simulink model "unicycle_b_point"  (R2025b)
settings: Solver=ode45  StartTime=0.0  StopTime=40  FixedStep=1e-4  MaxStep=0.01  RelTol=1e-3
settings Model: Creator=Cris  LastModifiedBy=Cris
settings DebuggingCC: UnderspecifiedInitializationDetection=Classic  MergeDetectMultiDrivingBlocksExec=none
settings ModelReferenceCC: PropagateSignalLabelsOutOfModel=off

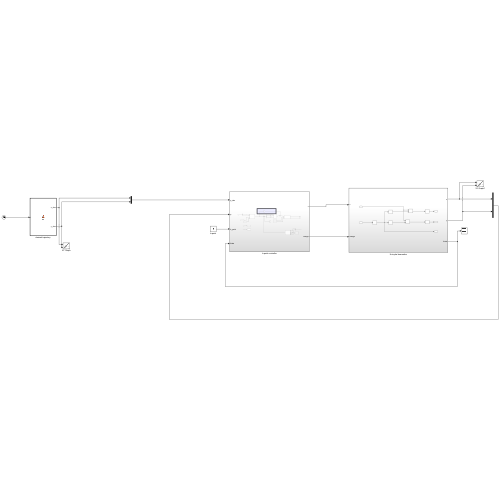
[thumbnail: Simulink's stored preview of the top-level diagram]
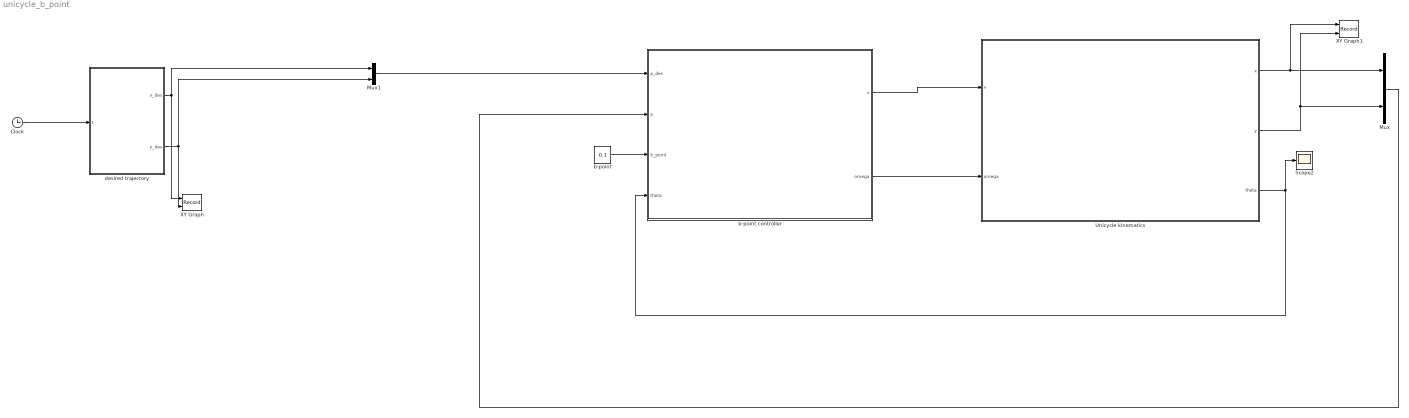
== system unicycle_b_point ==
  Clock : Clock
  Mux : Mux  Inputs=2
  Mux1 : Mux  Inputs=2
  Scope2 : Scope
      settings: ActiveDisplayYMinimum=-1  ActiveDisplayYMaximum=1
  Unicycle kinematics : Subsystem
  XY Graph : Record  NumPorts=2.0  FileSettingsInternal="{\"entries\":[{\"content\":{\"excelSettings\":{\"content\":{},\"type\":\"Streamout.ExcelSettings\"},\"parquetSettings\":{\"content\":{},\"type\":\"Streamout.ParquetSettings\"}},\"type\":\"Streamout.FileSettingStorage\",\"uuid\":\"\"}],\"packageUris\":[\"http:\\/\\/schema.mathworks.com\\/mf0\\/streamout_blocks\\/R2020a\"],\"version\":\"1.0\"}"  FrameSettings=[0, 0]  Layout=[1 1]  SignalsInternal="{\"entries\":[{\"content\":{\"signals\":[{\"content\":{\"blockPath\":[],\"dimensions\":[1],\"domain\":\"\",\"lineColor\":\"#a2142f\",\"plots\":[ 1 ],\"port\":1,\"sid\":[\"\"],\"signalID\":1,\"signalName\":\"desired trajectory:1\"},\"type\":\"RecordBlkView.Signal\",\"uuid\":\"\"},{\"content\":{\"blockPath\":[],\"dimensions\":[1],\"domain\":\"\",\"lineColor\":\"#139fff\",\"plots\":[ 1 ],\"port\":2,\"sid\":[\"\"],\"signalID\":2,\"signalName\":\"desired trajectory:2\"},\"type\":\"RecordBlkView.Signal\",\"uuid\":\"\"}]},\"type\":\"RecordBlkView.InputSignals\",\"uuid\":\"\"}],\"packageUris\":[\"http:\\/\\/schema.mathworks.com\\/mf0\\/streamout_blocks\\/R2020a\"],\"version\":\"1.0\"}"  VisualizationBindings="{\"xyplotplugin\":{\"info\":[{\"series\":[{\"bindingParametersList\":[{\"parameter\":\"X-Axis\",\"signalID\":1,\"signalName\":\"desired trajectory:1\"},{\"parameter\":\"Y-Axis\",\"signalID\":2,\"signalName\":\"desired trajectory:2\"}],\"seriesID\":0}],\"subplotID\":1}]}}"  CompatibilityTag=XY
  XY Graph1 : Record  NumPorts=2.0  FileSettingsInternal="{\"entries\":[{\"content\":{\"excelSettings\":{\"content\":{},\"type\":\"Streamout.ExcelSettings\"},\"parquetSettings\":{\"content\":{},\"type\":\"Streamout.ParquetSettings\"}},\"type\":\"Streamout.FileSettingStorage\",\"uuid\":\"\"}],\"packageUris\":[\"http:\\/\\/schema.mathworks.com\\/mf0\\/streamout_blocks\\/R2020a\"],\"version\":\"1.0\"}"  FrameSettings=[0, 0]  Layout=[1 1]  SignalsInternal="{\"entries\":[{\"content\":{\"signals\":[{\"content\":{\"blockPath\":[],\"dimensions\":[1],\"domain\":\"\",\"lineColor\":\"#a2142f\",\"plots\":[ 1 ],\"port\":1,\"sid\":[\"\"],\"signalID\":1,\"signalName\":\"Unicycle kinematics:1\"},\"type\":\"RecordBlkView.Signal\",\"uuid\":\"\"},{\"content\":{\"blockPath\":[],\"dimensions\":[1],\"domain\":\"\",\"lineColor\":\"#139fff\",\"plots\":[ 1 ],\"port\":2,\"sid\":[\"\"],\"signalID\":2,\"signalName\":\"Unicycle kinematics:2\"},\"type\":\"RecordBlkView.Signal\",\"uuid\":\"\"}]},\"type\":\"RecordBlkView.InputSignals\",\"uuid\":\"\"}],\"packageUris\":[\"http:\\/\\/schema.mathworks.com\\/mf0\\/streamout_blocks\\/R2020a\"],\"version\":\"1.0\"}"  VisualizationBindings="{\"xyplotplugin\":{\"info\":[{\"series\":[{\"bindingParametersList\":[{\"parameter\":\"X-Axis\",\"signalID\":1,\"signalName\":\"Unicycle kinematics:1\"},{\"parameter\":\"Y-Axis\",\"signalID\":2,\"signalName\":\"Unicycle kinematics:2\"}],\"seriesID\":0}],\"subplotID\":1}]}}"  CompatibilityTag=XY
  b-point : Constant  Value=0.1
  b-point controller : Subsystem
  desired trajectory : MATLAB Function  TreatAsAtomicUnit=on
  wires:
  Unicycle kinematics/1(x) -> XY Graph1/1, Mux/1
  Unicycle kinematics/2(y) -> XY Graph1/2, Mux/2
  Unicycle kinematics/3(theta) -> b-point controller/4(theta), Scope2/1
  desired trajectory/1(x_des) -> Mux1/1, XY Graph/1
  desired trajectory/2(y_des) -> Mux1/2, XY Graph/2
  Clock/1 -> desired trajectory/1(t)
  b-point controller/1(v) -> Unicycle kinematics/1(v)
  b-point controller/2(omega) -> Unicycle kinematics/2(omega)
  b-point/1 -> b-point controller/3(b_point)
  Mux1/1 -> b-point controller/1(p_des)
  Mux/1 -> b-point controller/2(p)

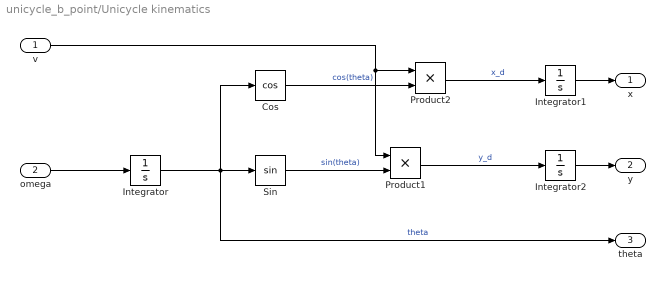
== system unicycle_b_point/Unicycle kinematics ==
  v : Inport
  omega : Inport  Port=2
  Cos : Trigonometry  Operator=cos
  Integrator : Integrator
  Integrator1 : Integrator
  Integrator2 : Integrator
  Product1 : Product
  Product2 : Product
  Sin : Trigonometry
  x : Outport
  y : Outport  Port=2
  theta : Outport  Port=3
  wires:
  omega/1 -> Integrator/1
  Integrator/1 -> theta/1, Cos/1, Sin/1  "theta"
  Cos/1 -> Product2/2  "cos(theta)"
  Sin/1 -> Product1/2  "sin(theta)"
  v/1 -> Product2/1, Product1/1
  Integrator1/1 -> x/1
  Product2/1 -> Integrator1/1  "x_d"
  Integrator2/1 -> y/1
  Product1/1 -> Integrator2/1  "y_d"

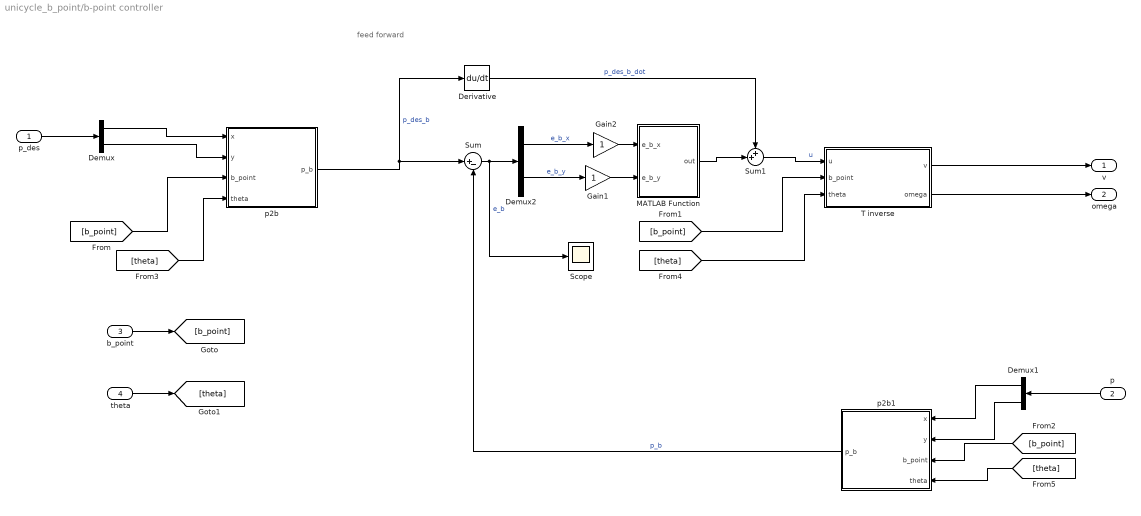
== system unicycle_b_point/b-point controller ==
  note: feed forward
  p_des : Inport
  p : Inport  Port=2
  b_point : Inport  Port=3
  theta : Inport  Port=4
  Demux : Demux  Outputs=2
  Demux1 : Demux  Outputs=2
  Demux2 : Demux  Outputs=2
  Derivative : Derivative
  Gain1 : Gain
  Gain2 : Gain
  MATLAB Function : MATLAB Function  TreatAsAtomicUnit=on
  Scope : Scope
      settings: ActiveDisplayYMinimum=-1  ActiveDisplayYMaximum=1
  Sum : Sum  Inputs=|+-
  Sum1 : Sum  Inputs=++|
  T inverse : MATLAB Function  TreatAsAtomicUnit=on
  p2b : MATLAB Function  TreatAsAtomicUnit=on
  p2b1 : MATLAB Function  TreatAsAtomicUnit=on
  v : Outport
  omega : Outport  Port=2
  wires:
  Derivative/1 -> Sum1/1  "p_des_b_dot"
  Sum1/1 -> T inverse/1(u)  "u"
  T inverse/1(v) -> v/1
  T inverse/2(omega) -> omega/1
  b_point/1 -> [b_point]
  [b_point] -> p2b/3(b_point)
  [b_point] -> T inverse/2(b_point)
  [b_point] -> p2b1/3(b_point)
  theta/1 -> [theta]
  [theta] -> p2b/4(theta)
  [theta] -> T inverse/3(theta)
  [theta] -> p2b1/4(theta)
  p2b1/1(p_b) -> Sum/2  "p_b"
  p2b/1(p_b) -> Derivative/1, Sum/1  "p_des_b"
  p_des/1 -> Demux/1
  Demux/1 -> p2b/1(x)
  Demux/2 -> p2b/2(y)
  p/1 -> Demux1/1
  Demux1/1 -> p2b1/1(x)
  Demux1/2 -> p2b1/2(y)
  Sum/1 -> Scope/1, Demux2/1  "e_b"
  Demux2/1 -> Gain2/1  "e_b_x"
  Demux2/2 -> Gain1/1  "e_b_y"
  Gain2/1 -> MATLAB Function/1(e_b_x)
  Gain1/1 -> MATLAB Function/2(e_b_y)
  MATLAB Function/1(out) -> Sum1/2

== matlab function unicycle_b_point/b-point controller/p2b1 ==
  data: x input; y input; p_b output; b_point input; theta input
function p_b = fcn(x, y, b_point, theta)

x_b = x + b_point * cos(theta);
y_b = y + b_point * sin(theta);

p_b = [x_b; y_b];

== matlab function unicycle_b_point/b-point controller/p2b ==
  data: x input; y input; p_b output; b_point input; theta input
function p_b = fcn(x, y, b_point, theta)

x_b = x + b_point * cos(theta);
y_b = y + b_point * sin(theta);

p_b = [x_b; y_b];

== matlab function unicycle_b_point/b-point controller/MATLAB Function ==
  data: e_b_x input size=1; out output; e_b_y input size=1
function out = fcn(e_b_x, e_b_y)

out = [e_b_x; e_b_y];

== matlab function unicycle_b_point/desired trajectory ==
  data: t input; x_des output; y_des output
function [x_des, y_des] = fcn(t)

% % configurable:
% radius = 5;
% omega_des = 0.2;
% 
% % desired trajectory
% x_des = -radius*cos(omega_des*t);
% y_des = -radius*sin(omega_des*t);


% % configurable:
% radius = 10;
% omega_des = 0.5;
% 
% % desired trajectory
% x_des = radius*cos(omega_des*t);
% y_des = radius*sin(omega_des*t);
% 


if t <= 10
    x_des = 10+t;
    y_des = 10;
elseif  t <= 20
    x_des = 20;
    y_des = 0+t;
elseif  t <= 30
    x_des = 40-t;
    y_des = 20;
elseif  t <= 40
    x_des = 10;
    y_des = 50-t;
else
    x_des = 100;
    y_des = 100;
end

== matlab function unicycle_b_point/b-point controller/T inverse ==
  data: u input size=2; b_point input size=1; v output size=1; omega output size=1; theta input size=1
function [v, omega] = fcn(u, b_point, theta)

% define matrix T inverse
T_inv = [cos(theta), sin(theta);
    -sin(theta)/b_point, cos(theta)/b_point];

% do calculation
res = T_inv * u;

% assign output
v = res(1, 1);
omega = res(2, 1);
